simulink model "Cessna_6DOF"  (Simulink 8.3)
settings: Solver=ode45  StartTime=0.0  StopTime=1000  RelTol=1e-3
values from neighbouring files (symbols this model uses):
  I_xx = 1285.31    [Initial_Cessna.m]
  I_yy = 1824.93    [Initial_Cessna.m]
  I_zz = 2666.893    [Initial_Cessna.m]
  p = 0    [Initial_Cessna.m]
  phi = 0    [Initial_Cessna.m]
  psi = 0    [Initial_Cessna.m]
  q = 0    [Initial_Cessna.m]
  r = 0    [Initial_Cessna.m]
  theta = alpha    [Initial_Cessna.m]
  v = V_trim*sin(beta)    [Initial_Cessna.m]
  w = V_trim*sin(alpha)*cos(beta)    [Initial_Cessna.m]
  x = 0    [Initial_Cessna.m]
  y = 0    [Initial_Cessna.m]
  z = 0    [Initial_Cessna.m]
libraries: aerolibobsolete x1, aerolibasang x1
settings Model: Creator=Pranav  LastModifiedBy=Pranav
settings OptimizationCC: ExpressionDepthLimit=2147483647
settings DebuggingCC: FcnCallInpInsideContextMsg=UseLocalSettings

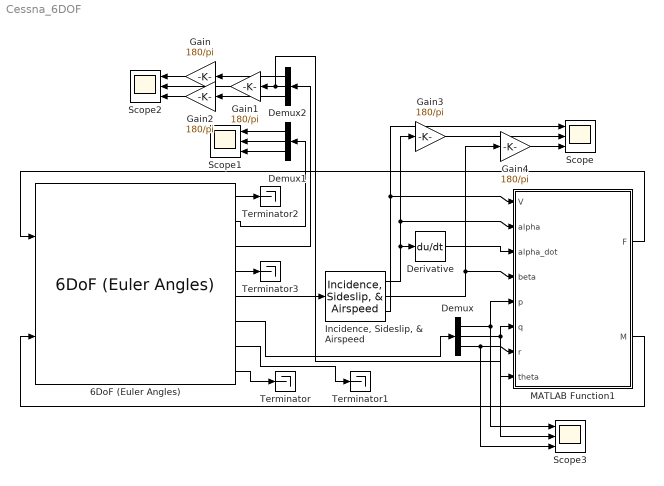
== system Cessna_6DOF ==
  6DoF (Euler Angles) : aerolibobsolete/6DoF (Euler Angles)  units=Metric (MKS)  mtype=Fixed  rep=Euler Angles  xme_0=[x y z]  Vm_0=[u v w]  eul_0=[phi theta psi]  pm_0=[p q r]  mass_0=m  mass_e=0.5  mass_f=2.0  inertia=diag([I_xx I_yy I_zz])  inertia_e=eye(3)  inertia_f=2*eye(3)  k_quat=1.0
  Demux : Demux  Outputs=3
  Demux1 : Demux  Outputs=3
  Demux2 : Demux  Outputs=3
  Derivative : Derivative
  Gain{,1..4} (5 alike) : Gain  Gain=180/pi
  "Incidence, Sideslip, & Airspeed" : aerolibasang/Incidence, Sideslip, & Airspeed
  MATLAB Function1 : MATLAB Function  TreatAsAtomicUnit=on
  Scope{,1..3} (4 alike) : Scope  NumInputPorts=3
      Scope settings: YMin=-5~-5~-5  YMax=5~5~5
      Scope1 settings: YMin=-5~-5~-5  YMax=5~5~5
      Scope2 settings: YMin=-5~-5~-5  YMax=5~5~5  SaveName=ScopeData2
      Scope3 settings: YMin=-5~-5~-5  YMax=5~5~5  SaveName=ScopeData3
  Terminator{,1..3} (4 alike) : Terminator
  wires:
  6DoF (Euler Angles)/5 -> "Incidence, Sideslip, & Airspeed"/1
  "Incidence, Sideslip, & Airspeed"/3 -> MATLAB Function1/1(V), Scope/1
  "Incidence, Sideslip, & Airspeed"/1 -> Derivative/1, MATLAB Function1/2(alpha), Gain3/1
  "Incidence, Sideslip, & Airspeed"/2 -> MATLAB Function1/4(beta), Gain4/1
  Derivative/1 -> MATLAB Function1/3(alpha_dot)
  Demux/1 -> MATLAB Function1/5(p), Scope3/1
  Demux/2 -> MATLAB Function1/6(q), Scope3/2
  Demux/3 -> MATLAB Function1/7(r), Scope3/3
  6DoF (Euler Angles)/6 -> Demux/1
  MATLAB Function1/1(F) -> 6DoF (Euler Angles)/1
  MATLAB Function1/2(M) -> 6DoF (Euler Angles)/2
  6DoF (Euler Angles)/7 -> Terminator1/1
  6DoF (Euler Angles)/8 -> Terminator/1
  6DoF (Euler Angles)/1 -> Terminator2/1
  6DoF (Euler Angles)/4 -> Terminator3/1
  Demux1/1 -> Scope1/1
  Demux1/2 -> Scope1/2
  Demux1/3 -> Scope1/3
  6DoF (Euler Angles)/2 -> Demux1/1
  Demux2/1 -> Gain/1
  Demux2/2 -> MATLAB Function1/8(theta), Gain1/1
  Demux2/3 -> Gain2/1
  6DoF (Euler Angles)/3 -> Demux2/1
  Gain/1 -> Scope2/1
  Gain1/1 -> Scope2/2
  Gain2/1 -> Scope2/3
  Gain3/1 -> Scope/2
  Gain4/1 -> Scope/3

== matlab function MATLAB Function1 ==
  data: V input double; F output double; alpha input double; alpha_dot input double; beta input double; p input double; q input double; r input double; theta input double; M output double
function [F, M] = FM_Cessna(V, alpha, alpha_dot, beta, p, q, r, theta)

g = 9.8;
rho = 1.225;

m = 1043.26;
C_bar = 1.493;
b = 10.911;
S_ref = 16.1651;

C_L_0 = 0.25;
C_L_alpha = 4.47;
C_L_q = 1.7;
C_L_delta_e = 0.3476;

% Ignore all other C_D derivatives excluding C_D_0
% Use C_D = C_D_0 + k*C_L^2

C_D_0 = 0.036;
k = 0.3;

C_Y_beta = -0.31;
C_Y_p = -0.037;
C_Y_r = 0.21;
C_Y_delta_a = 0;

C_l_beta = -0.089;
C_l_p = -0.47;
C_l_r = 0.096;
C_l_delta_a = -0.09;
C_l_delta_r = 0.0147;

C_M_0 = -0.02;
C_M_alpha = -1.8;
C_M_alpha_dot = -12.4;
C_M_delta_e = -1.28;

C_N_beta = 0.065;
C_N_p = -0.03;
C_N_r = -0.99;
C_N_delta_a = -0.0053;
C_N_delta_r = -0.0657;

% Use delta_e and thrust value from output of fsolve(@Trim_function)

delta_e = 0.0338;
delta_a = 0;
delta_r = 0;
thrust = 4219.6;

C_L = C_L_0 + C_L_alpha*alpha + C_L_q*(q*C_bar/(2*V)) + C_L_delta_e*delta_e;
C_D = C_D_0 + k*C_L^2;
C_Y = C_Y_beta*beta + C_Y_p*(p*b/(2*V)) + C_Y_r*(r*b/(2*V)) + C_Y_delta_a*delta_a;

C_l = C_l_beta*beta + C_l_p*(p*b/(2*V)) + C_l_r*(r*b/(2*V)) + C_l_delta_a*delta_a + C_l_delta_r*delta_r;
C_M = C_M_0 + C_M_alpha*alpha + C_M_alpha_dot*(alpha_dot*C_bar/(2*V)) + C_M_delta_e*delta_e;
C_N = C_N_beta*beta + C_N_p*(p*b/(2*V)) + C_N_r*(r*b/(2*V)) + C_N_delta_a*delta_a + C_N_delta_r*delta_r;

C_X = -C_D*cos(alpha) + C_L*sin(alpha);
C_Z = -C_D*sin(alpha) - C_L*cos(alpha);

F = zeros(3,1);
M = zeros(3,1);

q_bar = 0.5*rho*V*V;

F(1,1) = q_bar*S_ref*C_X - m*g*sin(theta) + thrust;
F(2,1) = q_bar*S_ref*C_Y;
F(3,1) = q_bar*S_ref*C_Z + m*g*cos(theta);

M(1,1) = q_bar*b*S_ref*C_l;
M(2,1) = q_bar*C_bar*S_ref*C_M;
M(3,1) = q_bar*b*S_ref*C_N;
